simulink model "my_vco"  (Simulink 7.3)
settings: Solver=ode23  StartTime=0.0  StopTime=10  RelTol=1e-3
libraries: commsynccomp2 x1
settings Model: Creator=sn00632  LastModifiedBy=sn00632  BufferReuse=off
settings DataIOCC: LimitDataPoints=off  SaveCompleteFinalSimState=on
settings OptimizationCC: OptimizeBlockIOStorage=off  BufferReuse=off  ExpressionFolding=off  LocalBlockOutputs=off

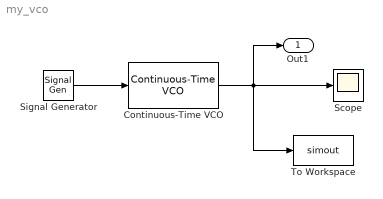
== system my_vco ==
  Continuous-Time VCO : commsynccomp2/Continuous-Time VCO  SystemSampleTime=-1  Ac=1  Fc=1  Kc=1  Ph=0
  Scope : Scope
      settings: TimeRange=10  YMin=-1  YMax=1  SaveName=yout  DataFormat=Array
  Signal Generator : SignalGenerator  WaveForm=sawtooth  Frequency=1000
  To Workspace : ToWorkspace  VariableName=simout  SampleTime=-1  SaveFormat=Array
  Out1 : Outport  OutDataType=fixdt(1, 16)  OutScaling=2^0
  wires:
  Continuous-Time VCO/1 -> To Workspace/1, Scope/1, Out1/1
  Signal Generator/1 -> Continuous-Time VCO/1
